simulink model "edge_trigger_outputEvent_eg"  (R2018a)
settings: Solver=VariableStepAuto  StartTime=0.0  StopTime=4  RelTol=1e-3
settings Model: Creator=86188  LastModifiedBy=86188

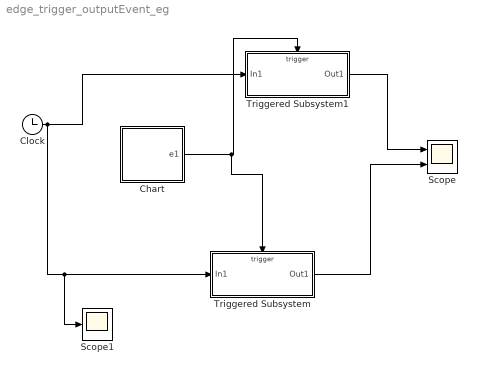
== system edge_trigger_outputEvent_eg ==
  Chart : Stateflow chart  TreatAsAtomicUnit=on
  Clock : Clock
  Scope : Scope  NumInputPorts=2
  Scope1 : Scope
  Triggered Subsystem : Subsystem  TreatAsAtomicUnit=on
  Triggered Subsystem1 : Subsystem  TreatAsAtomicUnit=on
  wires:
  Clock/1 -> Scope1/1, Triggered Subsystem/1(In1), Triggered Subsystem1/1(In1)
  Chart/1(e1) -> Triggered Subsystem/Trigger, Triggered Subsystem1/Trigger
  Triggered Subsystem1/1(Out1) -> Scope/1
  Triggered Subsystem/1(Out1) -> Scope/2

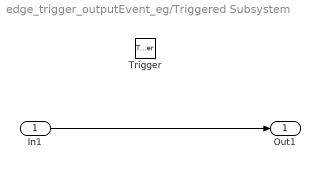
== system edge_trigger_outputEvent_eg/Triggered Subsystem ==
  In1 : Inport
  Trigger : TriggerPort  VariantControl=Variant
  Out1 : Outport
  wires:
  In1/1 -> Out1/1

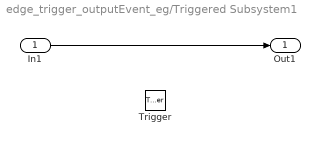
== system edge_trigger_outputEvent_eg/Triggered Subsystem1 ==
  In1 : Inport
  Trigger : TriggerPort  TriggerType=either  VariantControl=Variant
  Out1 : Outport
  wires:
  In1/1 -> Out1/1

== stateflow chart edge_trigger_outputEvent_eg/Chart ==
  state A
    du:a=1;
  state B
    en:send(e1);
    du:a=0;
  (default) -> A
  A -> B : [a==1]
  B -> A : [a==0]
  data: a local =0
  events: e1 output EITHER_EDGE_EVENT
